simulink model "BESSV6_Switchmodel"  (R2020b)
settings: Solver=FixedStepDiscrete  StartTime=0.0  StopTime=10  FixedStep=Tplant  RelTol=1e-3
undefined symbols (not defined in the file): D1, DCL_LSC_LCL_Trafo_NoSwitching, Delta, DiscIntNeverNeededParam, dq_to_abc_single_dual, ess, Idq_Dec_Signs_Fdbk_Ref, pwrsysVICtrl, pwrsysVSrc, systemBase, Tplant
libraries: powerlib x54, pwrsysBasic x15, powerlib_meascontrol x14, pwrsysTransf x7, simulink x3
settings Model: Creator=lokaladm_josephkb  LastModifiedBy=josephkb
settings DataIOCC: ReturnWorkspaceOutputs=off
settings SFSimCC: CustomCodeUndefinedFunction=UseInterfaceOnly

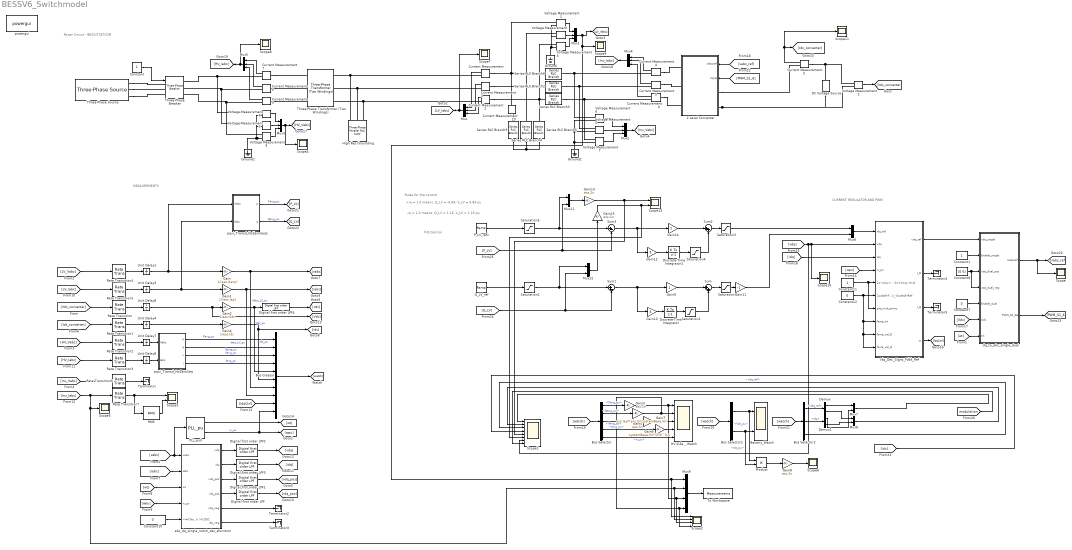
== system BESSV6_Switchmodel ==
  note: P-Q Control
  note: +iq = 1.0 means, Q_LV = -0.84, V_LV = 0.84 pu
  note: Rules for the control
  note: Power Circuit - BESS/STATCOM
  note: MEASUREMENTS
  note: CURRENT REGULATOR AND PWM
  note: -iq = 1.0 means, Q_LV = 1.16, V_LV = 1.16 pu
  2 Level Converter : Subsystem  AncestorBlock=pwrsysVSrc/DCL_LSC_LCL_Trafo_NoSwitching  mask(DCL + LSC + LCL + Trafo){Sn=ess.Sn, fn=systemBase.fn, Uhv_ab=systemBase.Vn, Uab=ess.Un, lf2=ess.LCL.l2, rf2=ess.LCL.r2, Lf1=ess.LCL.L1, Rf1=ess.LCL.R1, Cf=ess.LCL.Cf, Rc=ess.LCL.Rf, Cdc=ess.Cdc, Udc0=ess.Udc, Tsm=ess.Ts_control, Tstart=ess.DCVCont.Start}
      mask prompts: Sn "Rated apparent power [VA]"; fn "Rated frequency [Hz]"; Uhv_ab "Trafo HV rated line voltage [V]"; Uab "Trafo LV rated line voltage [V]"; lf2 "Trafo short-circuit inductance, lf2 [pu]"; rf2 "Trafo short-circuit resistance, rf2 [pu]"; Lf1 "Inverter side inductande, Lf1 [H]"; Rf1 "Inverter side parasitic resistance, Rf1 [Ohm]"; Cf "Shunt branch capacitance, Cf [F]"; Rc "Shunt branch damping resistance, Rc [Ohm]"; Cdc "DC-link shunt capacitance, Cdc [F]"; Udc0 "DC-link initial voltage [V]"; Tsm "Measurement sampling time [s]"; Tstart "Start time [s]"
      mask help:
      | DC Link + Line-side converter + LCL filter + Transformer
      |
      | DCL: current sources
      | 	Cdc: shunt capacitor of DC-link
      |
      | LSC: voltage source
      | 	fpwm: PWM frequency
      | LCL:
      | 	Lf1 + Rf1: inverter side reactor
      | 	Cf + Rc: shunt capacitor and damping resistor
      | 	Lf2 + Rf2: transformer short circuit inductance and resistance
      |
      | Transformer:	Y d1
      | 	HV: Y ungrounded
      | 	LV: delta
      |
      | High resistive grounding on LV side of tranformer (0.001W)
  Battery_Watch : Scope  NumInputPorts=2
  Bus Creator : BusCreator  Inputs=10
  Bus Selector : BusSelector  OutputSignals=Pavg_pu,Qavg_pu,Vavg_pu,Iavg_pu,w_pu
  Bus Selector1 : BusSelector  OutputSignals=Vdc_pu,Idc_pu
  Bus Selector2 : BusSelector  OutputSignals=IdqCtrl.Idq_ref,IdqCtrl.Idq,IdqCtrl.vdq_ref
  Constant : Constant
  Constant1 : Constant  SampleTime=ess.Ts_control
  Constant10 : Constant  Value=0  SampleTime=ess.Ts_control
  Constant11 : Constant  SampleTime=ess.Ts_control
  Constant12 : Constant  Value=0  SampleTime=ess.Ts_control
  Constant7 : Constant  Value=0  SampleTime=ess.Ts_control
  Constant9 : Constant  Value=[0 0]  SampleTime=ess.Ts_control
  Current Measurement{,1..10} (11 alike) : powerlib/Measurements/Current Measurement  PhasorSimulation=off  OutputType=Complex  PSBequivalent=0
  DC Voltage Source : powerlib/Electrical Sources/DC Voltage Source  Amplitude=ess.Udc  Measurements=None
  Demux : Demux  Outputs=2
  Demux1 : Demux  Outputs=2
  Digital first order LPF{,1..4} (5 alike) : pwrsysBasic/Digital first order LPF  Ts=ess.Ts_control  fcutout=ess.CurrCont.f_LPF_noise
      settings: SourceProductName=NTNU Power Systems
  Discrete-Time Integrator : DiscreteIntegrator  SampleTime=-1  ICPrevOutput=DiscIntNeverNeededParam  ICPrevScaledInput=DiscIntNeverNeededParam
  Discrete-Time Integrator1 : DiscreteIntegrator  SampleTime=-1  ICPrevOutput=DiscIntNeverNeededParam  ICPrevScaledInput=DiscIntNeverNeededParam
  Gain : Gain  Gain=1/(ess.Uanp)
  Gain1 : Gain  Gain=1/(ess.Iap)
  Gain10 : Gain  Gain=3
  Gain11 : Gain  Gain=-1
  Gain12 : Gain  Gain=3
  Gain{3,5,8,13,15} (5 alike) : Gain  Gain=ess.Sn
  Gain14 : Gain
  Gain2 : Gain  Gain=1/ess.Udc
  Gain4 : Gain  Gain=1/ess.Idc
  Gain6 : Gain  Gain=systemBase.Vn*(2/3)^0.5
  Gain7 : Gain  Gain=ess.Iap*(ess.Un/systemBase.Vn)
  Gain9 : Gain
  Ground : powerlib/Elements/Ground  LConnTagsString=a
  Ground1 : powerlib/Elements/Ground  LConnTagsString=a
  Ground2 : powerlib/Elements/Ground  LConnTagsString=a
  HV Side _ Watch : Scope  NumInputPorts=5
  High Res Grounding : powerlib/Elements/Three-Phase Parallel RLC Load  LConnTagsString=A|B|C  Configuration=Y (grounded)  NominalVoltage=ess.Un  Vabc=[1e3 1e3 1e3]  Vabcp=[1e3 1e3 1e3]  NominalFrequency=ess.Fn  UnbalancedPower=off  ActivePower=0.001  InductivePower=0  CapacitivePower=0  Pabc=[10e3 9e3 11e3]  QLabc=[100 90 110]  QCabc=[100 90 110]  Pabcp=[10e3 9e3 11e3]  QLabcp=[100 90 110]  QCabcp=[100 90 110]  Measurements=None  LoadType=constant Z
  Idq_Dec_Signs_Fdbk_Ref : Subsystem  AncestorBlock=pwrsysVICtrl/Idq_Dec_Signs_Fdbk_Ref  mask(Idq Controller - PI regulator with anti-windup){Ts=ess.Ts_control, fn=systemBase.fn, Kp=0.2, Ti=0.2/1, L=ess.CurrCont.x, PI_max=ess.CurrCont.PImax, PI_min=ess.CurrCont.PImin, TrafoPhaseComp=0}
      mask prompts: Ts "Sampling time [s]"; fn "Rated frequency: fn [Hz]"; Kp "Proportional gain: Kp [pu]"; Ti "Integral time: Ti [s]"; L "DQ decoupl. inductance: L [pu]"; PI_max "Maximum output [pu]"; PI_min "Minimum output [pu]"; TrafoPhaseComp "Transformer phase compensation [rad]"
      mask help:
      | Idq Controller
      | Discrete PI regulator with forward Euler approximation for the integrator.
      | Transfer function: 	Kp (1 + sTi) / (sTi)
      | The anti-windup freezes the integrator if the unlimited output of the PI goes beyond the limits.
      |
      | Phase compensation for transformer winding: PhaseTrafoComp
  Mux{,1..5} (6 alike) : Mux  Inputs=3
  Mux{6..8,11..12} (5 alike) : Mux  Inputs=2
  Mux9 : Mux
  PLL_pu3 : pwrsysBasic/PLL_pu  fn=systemBase.fn  Ts=ess.Ts_control  Kp_pll=90  Ki_pll=1200  Kd_pll=0  PLL_ini=60
      settings: SourceProductName=NTNU Power Systems
  P_LV_ref1 : simulink/Sources/Ramp  slope=0.5  start=2  InitialOutput=0
  Product : Product
  Q_LV_ref : simulink/Sources/Ramp  slope=0.2  start=15  InitialOutput=0
  RMS : powerlib_meascontrol/Measurements/RMS  TrueRMS=on  Freq=60  RMSInit=120  Ts=ess.Ts_control
  Rate Transition{,1..7} (8 alike) : RateTransition  OutPortSampleTime=ess.Ts_control
  Saturation{,1,3..4} (4 alike) : Saturate  UpperLimit=1  LowerLimit=-1
  Saturation2 : Saturate  UpperLimit=0.15  LowerLimit=-0.15
  Saturation5 : Saturate  LowerLimit=-0.4
  Scope{,4..11} (9 alike) : Scope
  Scope1 : Scope  NumInputPorts=8
  Scope13 : Scope  NumInputPorts=2
  Scope2 : Scope  NumInputPorts=4
  Scope3 : Scope  NumInputPorts=2
  Series RLC Branch2 : powerlib/Elements/Series RLC Branch  LConnTagsString=__new0  RConnTagsString=__new0  BranchType=RL  Resistance=ess.LCL.R1  Inductance=ess.LCL.L1  SetiL0=off  InitialCurrent=0  Capacitance=1e-6  Setx0=off  InitialVoltage=0  Measurements=None
  Series RLC Branch3 : powerlib/Elements/Series RLC Branch  LConnTagsString=__new0  RConnTagsString=__new0  BranchType=RL  Resistance=ess.LCL.R1  Inductance=ess.LCL.L1  SetiL0=off  InitialCurrent=0  Capacitance=1e-6  Setx0=off  InitialVoltage=0  Measurements=None
  Series RLC Branch4 : powerlib/Elements/Series RLC Branch  LConnTagsString=__new0  RConnTagsString=__new0  BranchType=RC  Resistance=ess.LCL.Rf  Inductance=1e-3  SetiL0=off  InitialCurrent=0  Capacitance=ess.LCL.Cf  Setx0=off  InitialVoltage=0  Measurements=None
  Series RLC Branch5 : powerlib/Elements/Series RLC Branch  LConnTagsString=__new0  RConnTagsString=__new0  BranchType=RC  Resistance=ess.LCL.Rf  Inductance=1e-3  SetiL0=off  InitialCurrent=0  Capacitance=ess.LCL.Cf  Setx0=off  InitialVoltage=0  Measurements=None
  Series RLC Branch6 : powerlib/Elements/Series RLC Branch  LConnTagsString=__new0  RConnTagsString=__new0  BranchType=RL  Resistance=ess.LCL.R1  Inductance=ess.LCL.L1  SetiL0=off  InitialCurrent=0  Capacitance=1e-6  Setx0=off  InitialVoltage=0  Measurements=None
  Series RLC Branch9 : powerlib/Elements/Series RLC Branch  LConnTagsString=__new0  RConnTagsString=__new0  BranchType=RC  Resistance=ess.LCL.Rf  Inductance=1e-3  SetiL0=off  InitialCurrent=0  Capacitance=ess.LCL.Cf  Setx0=off  InitialVoltage=0  Measurements=None
  Sum : Sum  Inputs=|++
  Sum1 : Sum  Inputs=|+-
  Sum2 : Sum  Inputs=|++
  Sum3 : Sum  Inputs=|+-
  Terminator{,2..5} (5 alike) : Terminator
  Three-Phase Transformer (Two Windings) : powerlib/Elements/Three-Phase Transformer (Two Windings)  Winding1Connection=Y  Winding2Connection=Delta (D1)  CoreType=Three single-phase transformers  SetSaturation=off  Hysteresis=off  DataFile='hysteresis'  SetInitialFlux=off  Measurements=None  UNITS=pu  NominalPower=[ess.Sn , ess.Fn]  Winding1=[systemBase.Vn ess.LCL.r2 ess.LCL.l2]  Winding2=[ess.Un ess.LCL.r2 ess.LCL.l2]  Rm=500.01  Lm=416.67  L0=0.5  Saturation=[0 0;0.0024 1;0.99999 1.2667]  InitialFluxes=[0.80002 -0.80002 0.7]  BreakLoop=off  DiscreteSolver=Trapezoidal iterative  DataType=off  TransfoNumber=1
  Three-Phase Breaker : powerlib/Elements/Three-Phase Breaker  InitialState=open  SwitchA=on  SwitchB=on  SwitchC=on  SwitchTimes="[1/60  5/60]"  External=on  BreakerResistance=0.01  SnubberResistance=1e6  SnubberCapacitance=1e9  Measurements=None
  Three-Phase Source : powerlib/Electrical Sources/Three-Phase Source  InternalConnection=Yg  VoltagePhases=off  Voltage=systemBase.Vn  PhaseAngle=0  Voltage_phases=[25e3 25e3 25e3]/sqrt(3)  PhaseAngles_phases=[0 -120 +120]  Frequency=systemBase.fn  NonIdealSource=on  SpecifyImpedance=off  Resistance=5e-3  Inductance=0.2e-6  ShortCircuitLevel=SCMVA  BaseVoltage=systemBase.Vn  XRratio=X_R  BusType=swing  Pref=10e3  Qref=0  Prefabc=[10e3, 10e3, 10e3]  Qrefabc=[0, 0, 0]  Qmin=-inf  Qmax=inf
  To Workspace : ToWorkspace  VariableName=Measurements  SaveFormat=Structure With Time  SampleTime=ess.Ts_control
  Unit Delay{1,3,7..8} (4 alike) : UnitDelay  InitialCondition=[0 0 0]  SampleTime=ess.Ts_control  HasFrameUpgradeWarning=on
  Unit Delay4 : UnitDelay  SampleTime=ess.Ts_control  HasFrameUpgradeWarning=on
  Unit Delay6 : UnitDelay  InitialCondition=1  SampleTime=ess.Ts_control  HasFrameUpgradeWarning=on
  Voltage Measurement{,1..9} (10 alike) : powerlib/Measurements/Voltage Measurement  PhasorSimulation=off  OutputType=Complex  PSBequivalent=0
  abc_dq_single_notch_dsc_sfunction : Subsystem  AncestorBlock=pwrsysTransf/abc_dq_single_notch_dsc_sfunction  mask(abc->dq with Matlab){Ts=ess.Ts_control, fn=2*systemBase.fn, zeta=ess.CurrCont.zeta}
      mask prompts: Ts "Sampling time [s]"; fn "Notch frequency [Hz]"; zeta "Zeta for notch filters"
      mask help:
      | To be done
      |
      | Max buffer size for DSC 500 samples
  dq_to_abc_single_dual : Subsystem  AncestorBlock=pwrsysVICtrl/dq_to_abc_single_dual  mask(Scaling of vdq ref and PWM gate generation){Ts=ess.Ts_control, Uabp=ess.Uabp}
      mask prompts: Ts "Sampling time [s]"; Uabp "Rated peak line voltage [V]"
      mask help:
      | Scales vdq_ref by: U_line_peak / Udc
      |
      | Add third harmonic to uabc_ref for overmodulation
  powergui : powerlib/powergui  Priority=1  SimulationMode=Discrete  SampleTime=Tplant  frequency=60  Iterations=50  frequencyindice=0  Pbase=100e6  ErrMax=1e-4  UnitsV=kV  UnitsW=MW  buscounter=0  FunctionMessages=off  echomessages=off  EnableUseOfTLC=off  CurrentSourceSwitches=off  DisableSnubberDevices=off  DisableRonSwitches=off  DisableVfSwitches=off  DisplayEquations=off  AutomaticDiscreteSolvers=off  SolverType=Tustin/Backward Euler (TBE)  Interpol=off  ExternalGateDelay=off  methode=off  Ts=100  x0status=blocks  SPID=on  SwTol=0  HookPort=off  NonlinearTolerance=0  nMaxIteration=15  ContinueOnMaxIteration=off  RestoreLinks=warning  ResistiveCurrentMeasurement=off  Frange=[0:2:500]  Ylog=off  Xlog=on  ShowGrid=off  save=off  variable=ZData  structure=0  ZoomFFT=off  StartTime=0.0  cycles=1  DisplayStyle=1  fundamental=60  FreqAxis=off  MaxFrequency=1000  frequencyindicesteady=1  RmsSteady=1  display=off
  pqui_Transd_NoZeroSeq : Subsystem  AncestorBlock=pwrsysBasic/pqui_Transd_NoZeroSeq  mask(u i p q transducer - No zero sequence){Sn=ess.Sn, Uanp=systemBase.Vn*(2/3)^0.5, Iap=ess.Iap*(ess.Un/systemBase.Vn)}
      mask prompts: Sn "Rated three-phase apparent power [VA]"; Uanp "Rated peak phase-to-groud voltage [V]"; Iap "Rated peak line current [A]"
      mask help:
      | Loosely based on Akagi 1984, but with Clarke Transformation for both the current and voltage
      | 	v  = (valpha^2 + vbeta^2)^0.5 / V_phase_peak
      | 	i   = (ialpha^2 + ibeta^2)^0.5 / I_line_peak
      | 	p  = 3/2 * (valpha ialpha +vbeta ibeta) / Sn
      | 	q  = 3/2 * (-valpha ibeta +vbeta ialpha) / Sn
  pqui_Transd_NoZeroSeq1 : Subsystem  AncestorBlock=pwrsysBasic/pqui_Transd_NoZeroSeq  mask(u i p q transducer - No zero sequence){Sn=ess.Sn, Uanp=systemBase.Vn*(2/3)^0.5, Iap=ess.Iap*(ess.Un/systemBase.Vn)}
      mask prompts: Sn "Rated three-phase apparent power [VA]"; Uanp "Rated peak phase-to-groud voltage [V]"; Iap "Rated peak line current [A]"
      mask help:
      | Loosely based on Akagi 1984, but with Clarke Transformation for both the current and voltage
      | 	v  = (valpha^2 + vbeta^2)^0.5 / V_phase_peak
      | 	i   = (ialpha^2 + ibeta^2)^0.5 / I_line_peak
      | 	p  = 3/2 * (valpha ialpha +vbeta ibeta) / Sn
      | 	q  = 3/2 * (-valpha ibeta +vbeta ialpha) / Sn
  wires:
  Voltage Measurement2/1 -> [Vdc_converter]
  Mux/1 -> Scope7/1, [LV_Iabc]
  Voltage Measurement/1 -> Mux1/2
  Voltage Measurement1/1 -> Mux1/1
  Voltage Measurement4/1 -> Mux1/3
  Mux1/1 -> Scope2/1, Mux9/1, Scope9/1, [LV_Vabc]
  Mux2/1 -> [Inv_Vabc]
  Voltage Measurement6/1 -> Mux2/1
  Voltage Measurement7/1 -> Mux2/3
  Voltage Measurement5/1 -> Mux2/2
  Current Measurement/1 -> Mux/1
  Current Measurement1/1 -> Mux/2
  Current Measurement2/1 -> Mux/3
  [iabc] -> abc_dq_single_notch_dsc_sfunction/2(iabc)
  pqui_Transd_NoZeroSeq/4(i) -> Bus Creator/4  "Iavg_pu"
  Digital first order LPF3/1 -> [idq]
  Digital first order LPF/1 -> [idq_pos]
  abc_dq_single_notch_dsc_sfunction/4(idq_pos) -> Digital first order LPF/1
  Digital first order LPF2/1 -> [vdq]
  Bus Creator/1 -> [watch]
  Unit Delay3/1 -> pqui_Transd_NoZeroSeq1/2(Iabc), Gain1/1
  abc_dq_single_notch_dsc_sfunction/1(vdq) -> Digital first order LPF2/1
  Digital first order LPF4/1 -> [vdc]
  abc_dq_single_notch_dsc_sfunction/2(idq) -> Digital first order LPF3/1
  [vabc] -> abc_dq_single_notch_dsc_sfunction/1(vabc), PLL_pu3/1
  Unit Delay8/1 -> pqui_Transd_NoZeroSeq/2(Iabc)
  abc_dq_single_notch_dsc_sfunction/3(vdq_pos) -> Digital first order LPF1/1
  Gain1/1 -> [iabc], Bus Creator/8  "Iabc_LV_pu"
  [wt] -> abc_dq_single_notch_dsc_sfunction/3(wt)
  [wpu] -> abc_dq_single_notch_dsc_sfunction/4(w_pu)
  Unit Delay6/1 -> [Vdc], Gain2/1
  Unit Delay7/1 -> pqui_Transd_NoZeroSeq/1(Vabc)
  abc_dq_single_notch_dsc_sfunction/6(idq_neg) -> Terminator3/1
  Gain2/1 -> Digital first order LPF4/1, Bus Creator/5  "Vdc_pu"
  Unit Delay1/1 -> pqui_Transd_NoZeroSeq1/1(Vabc), Gain/1
  PLL_pu3/1 -> [wt]
  abc_dq_single_notch_dsc_sfunction/5(vdq_neg) -> Terminator2/1
  Unit Delay4/1 -> Gain4/1
  Rate Transition2/1 -> Unit Delay7/1
  Rate Transition/1 -> Unit Delay6/1
  pqui_Transd_NoZeroSeq/1(p) -> Bus Creator/1  "Pavg_pu"
  PLL_pu3/2 -> Bus Creator/10, [wpu]  "w_pu"
  Rate Transition1/1 -> Unit Delay4/1
  [IdqCtrl] -> Bus Creator/9
  Digital first order LPF1/1 -> [vdq_pos]
  pqui_Transd_NoZeroSeq/3(v) -> Bus Creator/3  "Vavg_pu"
  Gain/1 -> [vabc], Bus Creator/7  "Vabc_LV_pu"
  Rate Transition3/1 -> Unit Delay8/1
  Gain4/1 -> [idc], Bus Creator/6  "Idc_pu"
  Constant10/1 -> abc_dq_single_notch_dsc_sfunction/5(<=0:Notch,>0:DSC)
  Rate Transition5/1 -> Unit Delay3/1
  Rate Transition4/1 -> Unit Delay1/1
  pqui_Transd_NoZeroSeq/2(q) -> Bus Creator/2  "Qavg_pu"
  Current Measurement3/1 -> Scope11/1, [Idc_converter]
  Voltage Measurement9/1 -> Mux3/3
  Voltage Measurement3/1 -> Mux3/2
  Voltage Measurement8/1 -> Mux3/1
  Constant/1 -> Three-Phase Breaker/1
  Current Measurement7/1 -> Mux5/1
  Current Measurement8/1 -> Mux5/2
  Mux5/1 -> Scope8/1, [HV_Iabc]
  Current Measurement9/1 -> Mux5/3
  Mux4/1 -> [Inv_Iabc]
  Current Measurement4/1 -> Mux4/1
  Current Measurement5/1 -> Mux4/2
  Current Measurement6/1 -> Mux4/3
  [Vdc_converter] -> Rate Transition/1
  [Idc_converter] -> Rate Transition1/1
  [HV_Vabc] -> Rate Transition2/1
  [HV_Iabc] -> Rate Transition3/1
  [LV_Vabc] -> Rate Transition4/1
  [LV_Iabc] -> Rate Transition5/1
  [Inv_Vabc] -> Rate Transition6/1
  [Inv_Iabc] -> Scope2/2, Mux9/2, Scope5/1, Rate Transition7/1
  Rate Transition6/1 -> Terminator/1
  Rate Transition7/1 -> RMS/1, Scope3/1
  [wpu] -> Idq_Dec_Signs_Fdbk_Ref/4(w_pu)
  Constant12/1 -> Idq_Dec_Signs_Fdbk_Ref/8(force_int), Idq_Dec_Signs_Fdbk_Ref/9(force_val_D), Idq_Dec_Signs_Fdbk_Ref/10(force_val_Q), Idq_Dec_Signs_Fdbk_Ref/6(1=decFrFbk_-0=decFrRef)
  Idq_Dec_Signs_Fdbk_Ref/3(I_Q) -> Terminator5/1
  Idq_Dec_Signs_Fdbk_Ref/4(m) -> [IdqCtrl]
  Constant11/1 -> Idq_Dec_Signs_Fdbk_Ref/7(pre_mult_errors), Idq_Dec_Signs_Fdbk_Ref/5(1=-wLiq,+wLid_-1=+wLiq,-wLid)
  [vdq] -> Scope1/7, Scope10/1, Idq_Dec_Signs_Fdbk_Ref/2(vdq)
  Constant9/1 -> dq_to_abc_single_dual/4(vdq_dual_neg), dq_to_abc_single_dual/3(vdq_dual_pos)
  Constant1/1 -> dq_to_abc_single_dual/2(Enable_single)
  Constant7/1 -> dq_to_abc_single_dual/5(Enable_dual)
  [wt] -> dq_to_abc_single_dual/7(wt)
  Idq_Dec_Signs_Fdbk_Ref/2(I_D) -> Terminator4/1
  [Vdc] -> dq_to_abc_single_dual/6(Udc)
  dq_to_abc_single_dual/1(Uabcref) -> Scope/1, [vabc_ref]
  [idq] -> Idq_Dec_Signs_Fdbk_Ref/3(idq)
  Idq_Dec_Signs_Fdbk_Ref/1(vdq_ref) -> dq_to_abc_single_dual/1(vdq_single)
  Mux6/1 -> Idq_Dec_Signs_Fdbk_Ref/1(idq_ref)
  [vabc_ref] -> 2 Level Converter/1(Vabcref)
  [watch] -> Bus Selector/1
  Bus Selector/1 -> Gain3/1  "<Pavg_pu>"
  Bus Selector/2 -> Gain5/1  "<Qavg_pu>"
  Bus Selector/3 -> Gain6/1  "<Vavg_pu>"
  Bus Selector/4 -> Gain7/1  "<Iavg_pu>"
  Bus Selector/5 -> HV Side _ Watch/5  "<w_pu>"
  Bus Selector1/1 -> Product/1, Battery_Watch/1  "<Vdc_pu>"
  Bus Selector1/2 -> Product/2, Battery_Watch/2  "<Idc_pu>"
  [watch] -> Bus Selector1/1
  [watch] -> Bus Selector2/1
  Bus Selector2/1 -> Demux/1  "<Idq_ref>"
  Bus Selector2/2 -> Demux1/1  "<Idq>"
  Bus Selector2/3 -> Scope1/3  "<vdq_ref>"
  Mux7/1 -> Scope1/1
  Mux8/1 -> Scope1/2
  Demux/1 -> Mux7/1
  Demux1/1 -> Mux7/2
  Demux/2 -> Mux8/1
  Demux1/2 -> Mux8/2
  [idc] -> Scope1/4
  RMS/1 -> Scope3/2
  Gain3/1 -> Scope2/3, Mux9/3, HV Side _ Watch/1
  Gain5/1 -> Scope2/4, Mux9/4, HV Side _ Watch/2
  Gain6/1 -> HV Side _ Watch/3
  Gain7/1 -> HV Side _ Watch/4
  Product/1 -> Gain8/1
  Gain8/1 -> Scope6/1
  Mux3/1 -> Scope4/1, [HV_Vabc]
  pqui_Transd_NoZeroSeq1/1(p) -> [P_LV]  "Pavg_pu"
  Gain10/1 -> Discrete-Time Integrator/1
  Discrete-Time Integrator/1 -> Saturation1/1
  Sum/1 -> Saturation/1
  Gain9/1 -> Sum/1
  Saturation1/1 -> Sum/2
  Sum1/1 -> Gain10/1, Gain9/1
  Q_LV_ref/1 -> Saturation2/1
  Mux12/1 -> Gain15/1
  Saturation/1 -> Gain11/1
  Gain11/1 -> Mux6/2
  Saturation2/1 -> Mux12/1, Sum1/1
  pqui_Transd_NoZeroSeq1/2(q) -> [Q_LV]  "Qavg_pu"
  [Q_LV] -> Mux12/2, Sum1/2
  Sum2/1 -> Saturation3/1
  Sum3/1 -> Gain12/1, Gain14/1
  Gain14/1 -> Sum2/1
  Mux11/1 -> Gain13/1
  Gain12/1 -> Discrete-Time Integrator1/1
  Discrete-Time Integrator1/1 -> Saturation4/1
  [P_LV] -> Sum3/2, Mux11/2
  P_LV_ref1/1 -> Saturation5/1
  Saturation5/1 -> Mux11/1, Sum3/1
  Saturation4/1 -> Sum2/2
  Saturation3/1 -> Mux6/1
  Gain13/1 -> Scope1/5, Scope13/1
  Gain15/1 -> Scope1/6, Scope13/2
  [modulation] -> Scope1/8
  dq_to_abc_single_dual/2(PWM_S1_S6) -> [PWM_S1_6]
  [PWM_S1_6] -> 2 Level Converter/2(PWM)
  Mux9/1 -> To Workspace/1
  connections:
  Voltage Measurement3/LConn1 -- Current Measurement8/RConn1 -- Three-Phase Breaker/RConn2
  Three-Phase Breaker/RConn1 -- Current Measurement7/RConn1 -- Voltage Measurement8/LConn1
  Voltage Measurement9/LConn1 -- Current Measurement9/RConn1 -- Three-Phase Breaker/RConn3
  Current Measurement/RConn1 -- Three-Phase Transformer (Two Windings)/RConn1 -- High Res Grounding/LConn1
  Series RLC Branch6/LConn1 -- Voltage Measurement1/LConn1 -- Current Measurement/LConn1 -- Current Measurement10/LConn1
  Series RLC Branch4/LConn1 -- Series RLC Branch2/LConn1 -- Current Measurement1/LConn1 -- Voltage Measurement/LConn1
  Series RLC Branch5/LConn1 -- Series RLC Branch3/LConn1 -- Current Measurement2/LConn1 -- Voltage Measurement4/LConn1
  Current Measurement1/RConn1 -- Three-Phase Transformer (Two Windings)/RConn2 -- High Res Grounding/LConn2
  Current Measurement2/RConn1 -- Three-Phase Transformer (Two Windings)/RConn3 -- High Res Grounding/LConn3
  Voltage Measurement2/LConn1 -- Current Measurement3/LConn1 -- DC Voltage Source/RConn1
  2 Level Converter/LConn2 -- DC Voltage Source/LConn1 -- Voltage Measurement2/LConn2
  Ground/LConn1 -- Voltage Measurement4/LConn2 -- Voltage Measurement/LConn2 -- Voltage Measurement1/LConn2
  Series RLC Branch6/RConn1 -- Current Measurement4/RConn1 -- Voltage Measurement6/LConn1
  Series RLC Branch2/RConn1 -- Current Measurement5/RConn1 -- Voltage Measurement5/LConn1
  Series RLC Branch3/RConn1 -- Current Measurement6/RConn1 -- Voltage Measurement7/LConn1
  2 Level Converter/LConn1 -- Current Measurement3/RConn1
  Voltage Measurement9/LConn2 -- Ground1/LConn1 -- Voltage Measurement3/LConn2 -- Voltage Measurement8/LConn2
  Three-Phase Source/RConn1 -- Three-Phase Breaker/LConn1
  Three-Phase Source/RConn2 -- Three-Phase Breaker/LConn2
  Three-Phase Source/RConn3 -- Three-Phase Breaker/LConn3
  Current Measurement7/LConn1 -- Three-Phase Transformer (Two Windings)/LConn1
  Current Measurement8/LConn1 -- Three-Phase Transformer (Two Windings)/LConn2
  Current Measurement9/LConn1 -- Three-Phase Transformer (Two Windings)/LConn3
  Series RLC Branch5/RConn1 -- Series RLC Branch9/RConn1 -- Series RLC Branch4/RConn1
  Voltage Measurement6/LConn2 -- Voltage Measurement5/LConn2 -- Voltage Measurement7/LConn2 -- Ground2/LConn1
  Current Measurement4/LConn1 -- 2 Level Converter/RConn1
  Current Measurement5/LConn1 -- 2 Level Converter/RConn2
  Current Measurement6/LConn1 -- 2 Level Converter/RConn3
  Current Measurement10/RConn1 -- Series RLC Branch9/LConn1

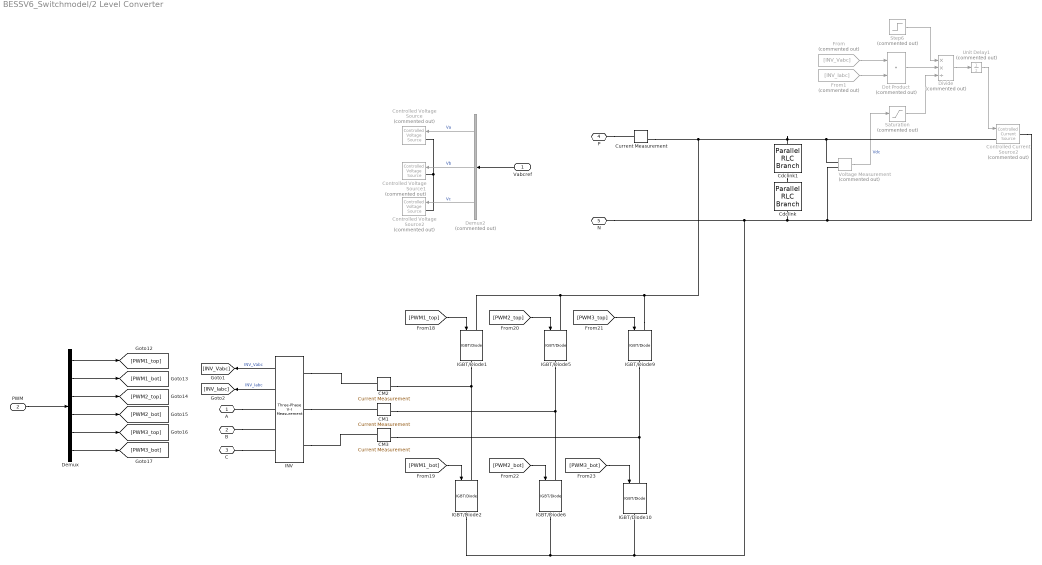
== system BESSV6_Switchmodel/2 Level Converter ==
  Vabcref : Inport
  PWM : Inport  Port=2
  CM1 : powerlib/Measurements/Current Measurement  PhasorSimulation=off  OutputType=Complex  PSBequivalent=0
  CM2 : powerlib/Measurements/Current Measurement  PhasorSimulation=off  OutputType=Complex  PSBequivalent=0
  CM3 : powerlib/Measurements/Current Measurement  PhasorSimulation=off  OutputType=Complex  PSBequivalent=0
  Cdclink : powerlib/Elements/Parallel RLC Branch  LConnTagsString=a  RConnTagsString=__new0  BranchType=RC  Resistance=1e6  Inductance=0  SetiL0=off  InitialCurrent=0  Capacitance=Cdc  Setx0=on  InitialVoltage=Udc0  Measurements=None
  Cdclink1 : powerlib/Elements/Parallel RLC Branch  LConnTagsString=a  RConnTagsString=__new0  BranchType=R  Resistance=1e-3  Inductance=0  SetiL0=off  InitialCurrent=0  Capacitance=Cdc  Setx0=on  InitialVoltage=Udc0  Measurements=None
  Controlled Current Source2 : powerlib/Electrical Sources/Controlled Current Source  Commented=on  Initialize=on  Source_Type=DC  Amplitude=0  Phase=0  Frequency=50  Measurements=None
  Controlled Voltage Source : powerlib/Electrical Sources/Controlled Voltage Source  Commented=on  Initialize=on  Source_Type=AC  Amplitude=Uab*(2/3)^0.5  Phase=30  Frequency=fn  Measurements=None
  Controlled Voltage Source1 : powerlib/Electrical Sources/Controlled Voltage Source  Commented=on  Initialize=on  Source_Type=AC  Amplitude=Uab*(2/3)^0.5  Phase=30-120  Frequency=fn  Measurements=None
  Controlled Voltage Source2 : powerlib/Electrical Sources/Controlled Voltage Source  Commented=on  Initialize=on  Source_Type=AC  Amplitude=Uab*(2/3)^0.5  Phase=30+120  Frequency=fn  Measurements=None
  Current Measurement : powerlib/Measurements/Current Measurement  PhasorSimulation=off  OutputType=Complex  PSBequivalent=0
  Demux : Demux  Outputs=6
  Demux2 : Demux  Commented=on  Outputs=3
  Divide : Product  Commented=on  Inputs=**/
  Dot Product : DotProduct  Commented=on  InputSameDT=on  OutDataTypeStr=Inherit: Inherit via internal rule
  From : From  Commented=on  GotoTag=INV_Vabc
  From1 : From  Commented=on  GotoTag=INV_Iabc
  IGBT/Diode{1..2,5..6,9..10} (6 alike) : powerlib/Power Electronics/IGBT//Diode  Ron=1e-3  Rs=1e5  Cs=inf  Measurements=off
  INV : powerlib/Measurements/Three-Phase V-I Measurement  VoltageMeasurement=phase-to-ground  SetLabelV=off  LabelV=vconv  Vpu=off  VpuLL=off  CurrentMeasurement=yes  SetLabelI=off  LabelI=iconv  Ipu=off  Pbase=sn  Vbase=uab  OutputType=Complex  PhasorSimulation=off  PSBequivalent=0
  Saturation : Saturate  Commented=on  UpperLimit=10*Uab*sqrt(2/3)  LowerLimit=0.01*Uab*sqrt(2/3)
  Step6 : Step  Commented=on  Time=Tstart  SampleTime=Tsm
  Unit Delay1 : UnitDelay  Commented=on  SampleTime=Tsm  HasFrameUpgradeWarning=on
  Voltage Measurement : powerlib/Measurements/Voltage Measurement  Commented=on  PhasorSimulation=off  OutputType=Magnitude  PSBequivalent=0
  A : PMIOPort  Side=Right
  B : PMIOPort  Port=2  Side=Right
  C : PMIOPort  Port=3  Side=Right
  P : PMIOPort  Port=4  Side=Left
  N : PMIOPort  Port=5  Side=Left
  wires:
  Step6/1 -> Divide/1
  Unit Delay1/1 -> Controlled Current Source2/1
  From1/1 -> Dot Product/2
  From/1 -> Dot Product/1
  Divide/1 -> Unit Delay1/1
  Dot Product/1 -> Divide/2
  Saturation/1 -> Divide/3
  Voltage Measurement/1 -> Saturation/1  "Vdc"
  Demux2/3 -> Controlled Voltage Source2/1  "Vc"
  Demux2/2 -> Controlled Voltage Source1/1  "Vb"
  Demux2/1 -> Controlled Voltage Source/1  "Va"
  Vabcref/1 -> Demux2/1
  INV/2 -> [INV_Iabc]  "INV_Iabc"
  INV/1 -> [INV_Vabc]  "INV_Vabc"
  Demux/6 -> [PWM3_bot]
  Demux/1 -> [PWM1_top]
  Demux/2 -> [PWM1_bot]
  Demux/3 -> [PWM2_top]
  Demux/4 -> [PWM2_bot]
  Demux/5 -> [PWM3_top]
  PWM/1 -> Demux/1
  [PWM2_top] -> IGBT/Diode5/1
  [PWM3_bot] -> IGBT/Diode10/1
  [PWM3_top] -> IGBT/Diode9/1
  [PWM2_bot] -> IGBT/Diode6/1
  [PWM1_bot] -> IGBT/Diode2/1
  [PWM1_top] -> IGBT/Diode1/1
  connections:
  P/RConn1 -- Current Measurement/LConn1
  IGBT/Diode9/LConn1 -- Current Measurement/RConn1 -- Cdclink1/LConn1 -- Voltage Measurement/LConn1 -- Controlled Current Source2/LConn1 -- IGBT/Diode5/LConn1 -- IGBT/Diode1/LConn1
  IGBT/Diode10/RConn1 -- N/RConn1 -- Cdclink/RConn1 -- Controlled Current Source2/RConn1 -- Voltage Measurement/LConn2 -- IGBT/Diode6/RConn1 -- IGBT/Diode2/RConn1
  Controlled Voltage Source1/LConn1 -- Controlled Voltage Source/LConn1 -- Controlled Voltage Source2/LConn1
  C/RConn1 -- INV/RConn3
  B/RConn1 -- INV/RConn2
  A/RConn1 -- INV/RConn1
  Cdclink1/RConn1 -- Cdclink/LConn1
  CM1/RConn1 -- IGBT/Diode6/LConn1 -- IGBT/Diode5/RConn1
  CM3/RConn1 -- IGBT/Diode10/LConn1 -- IGBT/Diode9/RConn1
  CM2/RConn1 -- IGBT/Diode2/LConn1 -- IGBT/Diode1/RConn1
  INV/LConn1 -- CM2/LConn1
  INV/LConn2 -- CM1/LConn1
  INV/LConn3 -- CM3/LConn1

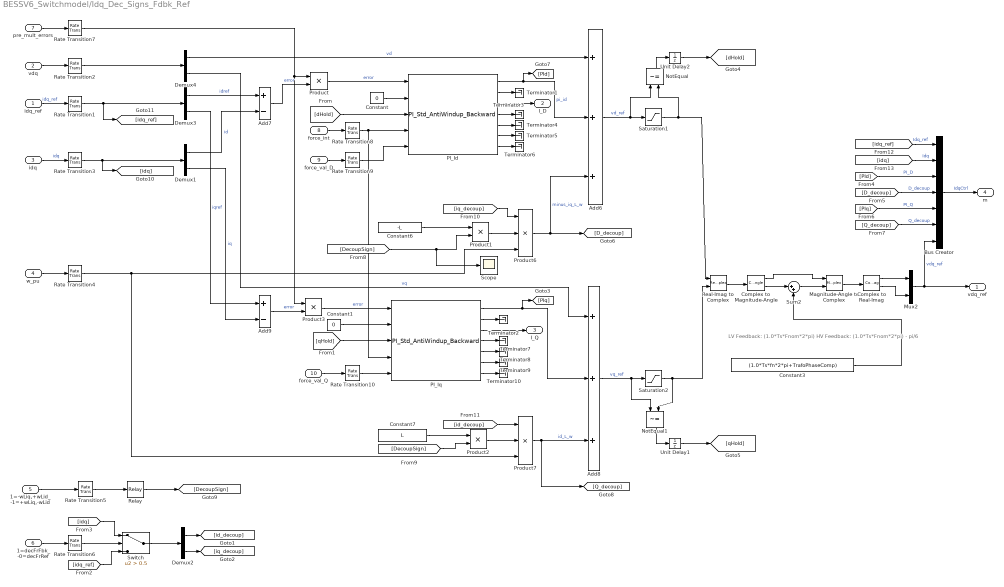
== system BESSV6_Switchmodel/Idq_Dec_Signs_Fdbk_Ref ==
  note: LV Feedback: (1.0*Ts*Fnom*2*pi)
      | HV Feedback: (1.0*Ts*Fnom*2*pi) - pi/6
  idq_ref : Inport
  vdq : Inport  Port=2
  idq : Inport  Port=3
  w_pu : Inport  Port=4
  1=-wLiq,+wLid_-1=+wLiq,-wLid : Inport  Port=5
  1=decFrFbk_-0=decFrRef : Inport  Port=6
  pre_mult_errors : Inport  Port=7
  force_int : Inport  Port=8
  force_val_D : Inport  Port=9
  force_val_Q : Inport  Port=10
  Add6 : Sum  Inputs=+++
  Add7 : Sum  Inputs=+-
  Add8 : Sum  Inputs=+++
  Add9 : Sum  Inputs=+-
  Bus Creator : BusCreator  Inputs=7
  Complex to Magnitude-Angle : ComplexToMagnitudeAngle
  Complex to Real-Imag : ComplexToRealImag
  Constant : Constant  Value=0  SampleTime=Ts
  Constant1 : Constant  Value=0  SampleTime=Ts
  Constant3 : Constant  Value=(1.0*Ts*fn*2*pi+TrafoPhaseComp)  SampleTime=Ts
  Constant6 : Constant  Value=-L  SampleTime=Ts
  Constant7 : Constant  Value=L  SampleTime=Ts
  Demux{1..4} (4 alike) : Demux  Outputs=2
  Magnitude-Angle to Complex : MagnitudeAngleToComplex
  Mux2 : Mux  Inputs=2
  NotEqual : RelationalOperator  Operator=~=  OutDataTypeStr=boolean  RndMeth=Nearest
  NotEqual1 : RelationalOperator  Operator=~=  OutDataTypeStr=boolean  RndMeth=Nearest
  PI_Id : pwrsysBasic/PI_Std_AntiWindup_Backward  Ts=Ts  Kg=Kp  Kp=1  Ti=Ti  outMax=PI_max  outMin=PI_min
      link override S-Function Builder: Parameters=Ts,Kg,Kp,Ti,outMax,outMin  FunctionName=pi_std_antiwindup
      settings: SourceProductName=NTNU Power Systems
  PI_Iq : pwrsysBasic/PI_Std_AntiWindup_Backward  Ts=Ts  Kg=Kp  Kp=1  Ti=Ti  outMax=PI_max  outMin=PI_min
      settings: SourceProductName=NTNU Power Systems
  Product : Product
  Product1 : Product  RndMeth=Zero
  Product2 : Product  RndMeth=Zero
  Product3 : Product
  Product6 : Product  Inputs=3  RndMeth=Zero
  Product7 : Product  Inputs=3  RndMeth=Zero
  Rate Transition1 : RateTransition  InitialCondition=[0 0]  OutPortSampleTime=Ts
  Rate Transition{6..10} (5 alike) : RateTransition  OutPortSampleTime=Ts
  Rate Transition2 : RateTransition  InitialCondition=[0 0]  OutPortSampleTime=Ts
  Rate Transition3 : RateTransition  InitialCondition=[0 0]  OutPortSampleTime=Ts
  Rate Transition4 : RateTransition  InitialCondition=1  OutPortSampleTime=Ts
  Rate Transition5 : RateTransition  InitialCondition=1  OutPortSampleTime=Ts
  Real-Imag to Complex : RealImagToComplex
  Relay : Relay  OnSwitchValue=0  OffSwitchValue=-0.1  OffOutputValue=-1
  Saturation1 : Saturate  UpperLimit=PI_max  LowerLimit=PI_min
  Saturation2 : Saturate  UpperLimit=PI_max  LowerLimit=PI_min
  Scope : Scope
  Sum2 : Sum  Inputs=|++
  Switch : Switch  Criteria=u2 > Threshold  Threshold=0.5
  Terminator{1..10} (10 alike) : Terminator
  Unit Delay1 : UnitDelay  SampleTime=Ts  HasFrameUpgradeWarning=on
  Unit Delay2 : UnitDelay  SampleTime=Ts  HasFrameUpgradeWarning=on
  vdq_ref : Outport
  I_D : Outport  Port=2
  I_Q : Outport  Port=3
  m : Outport  Port=4
  wires:
  Rate Transition10/1 -> PI_Iq/5
  Rate Transition9/1 -> PI_Id/5
  Rate Transition8/1 -> PI_Id/4, PI_Iq/4
  Rate Transition7/1 -> Product/1, Product3/1
  Rate Transition6/1 -> Switch/2
  Rate Transition5/1 -> Relay/1
  Rate Transition4/1 -> Product6/3, Product7/3
  Rate Transition3/1 -> [idq], Demux1/1
  Rate Transition1/1 -> Demux3/1, [idq_ref]
  Rate Transition2/1 -> Demux4/1
  Constant1/1 -> PI_Iq/2
  PI_Iq/1 -> [PIq], Add8/2
  PI_Iq/3 -> I_Q/1
  PI_Iq/7 -> Terminator10/1
  PI_Iq/6 -> Terminator9/1
  PI_Iq/5 -> Terminator8/1
  PI_Iq/4 -> Terminator7/1
  PI_Iq/2 -> Terminator2/1
  PI_Id/7 -> Terminator6/1
  PI_Id/6 -> Terminator5/1
  PI_Id/5 -> Terminator4/1
  PI_Id/4 -> Terminator3/1
  PI_Id/2 -> Terminator1/1
  Constant/1 -> PI_Id/2
  PI_Id/3 -> I_D/1
  pre_mult_errors/1 -> Rate Transition7/1
  Add7/1 -> Product/2  "error"
  Add9/1 -> Product3/2  "error"
  force_val_Q/1 -> Rate Transition10/1
  force_val_D/1 -> Rate Transition9/1
  force_int/1 -> Rate Transition8/1
  [idq] -> Bus Creator/2  "Idq"
  [idq_ref] -> Bus Creator/1  "Idq_ref"
  [id_decoup] -> Product7/1
  [iq_decoup] -> Product6/1
  [idq] -> Switch/1
  Switch/1 -> Demux2/1
  Demux2/1 -> [id_decoup]
  1=decFrFbk_-0=decFrRef/1 -> Rate Transition6/1
  Demux2/2 -> [iq_decoup]
  [idq_ref] -> Switch/3
  [DecoupSign] -> Product2/2
  Product2/1 -> Product7/2
  Product1/1 -> Product6/2
  [DecoupSign] -> Scope/1, Product1/2
  1=-wLiq,+wLid_-1=+wLiq,-wLid/1 -> Rate Transition5/1
  Relay/1 -> [DecoupSign]
  [qHold] -> PI_Iq/3
  [dHold] -> PI_Id/3
  Unit Delay1/1 -> [qHold]
  Unit Delay2/1 -> [dHold]
  NotEqual1/1 -> Unit Delay1/1
  Saturation2/1 -> Real-Imag to Complex/2, NotEqual1/2
  NotEqual/1 -> Unit Delay2/1
  Saturation1/1 -> Real-Imag to Complex/1, NotEqual/2
  [Q_decoup] -> Bus Creator/6  "Q_decoup"
  Bus Creator/1 -> m/1  "IdqCtrl"
  [PIq] -> Bus Creator/5  "PI_Q"
  [D_decoup] -> Bus Creator/4  "D_decoup"
  [PId] -> Bus Creator/3  "PI_D"
  Complex to Real-Imag/2 -> Mux2/2
  Complex to Real-Imag/1 -> Mux2/1
  Constant3/1 -> Sum2/2
  Sum2/1 -> Magnitude-Angle to Complex/2
  Complex to Magnitude-Angle/2 -> Sum2/1
  Complex to Magnitude-Angle/1 -> Magnitude-Angle to Complex/1
  Real-Imag to Complex/1 -> Complex to Magnitude-Angle/1
  Magnitude-Angle to Complex/1 -> Complex to Real-Imag/1
  Demux3/2 -> Add9/1  "iqref"
  Demux3/1 -> Add7/1  "idref"
  idq_ref/1 -> Rate Transition1/1  "idq_ref"
  Add6/1 -> Saturation1/1, NotEqual/1  "vd_ref"
  Add8/1 -> Saturation2/1, NotEqual1/1  "vq_ref"
  vdq/1 -> Rate Transition2/1
  idq/1 -> Rate Transition3/1  "idq"
  Mux2/1 -> vdq_ref/1, Bus Creator/7  "vdq_ref"
  Demux4/2 -> Add8/1  "vq"
  Product6/1 -> [D_decoup], Add6/3  "minus_iq_L_w"
  Demux1/2 -> Add9/2  "iq"
  Product/1 -> PI_Id/1  "error"
  Demux4/1 -> Add6/1  "vd"
  Product7/1 -> Add8/3, [Q_decoup]  "id_L_w"
  Demux1/1 -> Add7/2  "id"
  Constant7/1 -> Product2/1
  Constant6/1 -> Product1/1
  PI_Id/1 -> [PId], Add6/2  "pi_id"
  Product3/1 -> PI_Iq/1  "error"
  w_pu/1 -> Rate Transition4/1

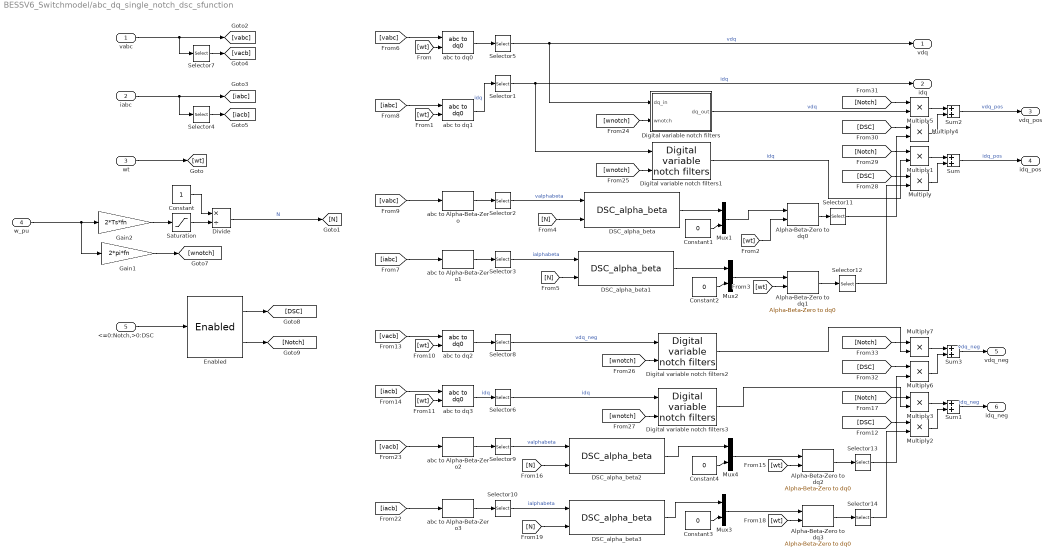
== system BESSV6_Switchmodel/abc_dq_single_notch_dsc_sfunction ==
  vabc : Inport
  iabc : Inport  Port=2
  wt : Inport  Port=3
  w_pu : Inport  Port=4
  <=0:Notch,>0:DSC : Inport  Port=5
  Alpha-Beta-Zero to dq{0..3} (4 alike) : powerlib_meascontrol/Transformations/Alpha-Beta-Zero to dq0  Alignment=90 degrees behind phase A axis
  Constant : Constant
  Constant{1..4} (4 alike) : Constant  Value=0
  DSC_alpha_beta{,1..3} (4 alike) : pwrsysBasic/DSC_alpha_beta  nmax=1/(2*Ts*fn*0.8)
      settings: SourceProductName=NTNU Power Systems
  Digital variable notch filters : Subsystem
  Digital variable notch filters1 : pwrsysTransf/abc_dq_single_notch_dsc_sfunction/Digital variable notch filters  SystemSampleTime=-1  VariantActivationTime=update diagram  Latency=0  AutoFrameSizeCalculation=off
      settings: SourceProductName=NTNU Power Systems
  Digital variable notch filters2 : pwrsysTransf/abc_dq_single_notch_dsc_sfunction/Digital variable notch filters  SystemSampleTime=-1  VariantActivationTime=update diagram  Latency=0  AutoFrameSizeCalculation=off
      settings: SourceProductName=NTNU Power Systems
  Digital variable notch filters3 : pwrsysTransf/abc_dq_single_notch_dsc_sfunction/Digital variable notch filters  SystemSampleTime=-1  VariantActivationTime=update diagram  Latency=0  AutoFrameSizeCalculation=off
      settings: SourceProductName=NTNU Power Systems
  Divide : Product  Inputs=*/
  Enabled : pwrsysBasic/Enabled
      settings: SourceProductName=NTNU Power Systems
  Gain1 : Gain  Gain=2*pi*fn
  Gain2 : Gain  Gain=2*Ts*fn
  Multiply{,1..7} (8 alike) : Product
  Mux{1..4} (4 alike) : Mux  Inputs=[2 1]
  Saturation : Saturate  UpperLimit=inf  LowerLimit=0.000001
  Selector{1..3,5..6,8..14} (12 alike) : Selector  InputPortWidth=3  IndexOptions=Index vector (dialog)  Indices=[1 2]  OutputSizes=1
  Selector4 : Selector  InputPortWidth=3  IndexOptions=Index vector (dialog)  Indices=[1 3 2]  OutputSizes=1
  Selector7 : Selector  InputPortWidth=3  IndexOptions=Index vector (dialog)  Indices=[1 3 2]  OutputSizes=1
  Sum{,1..3} (4 alike) : Sum
  abc to Alpha-Beta-Zero{,1..3} (4 alike) : powerlib_meascontrol/Transformations/abc to Alpha-Beta-Zero
  abc to dq{0..3} (4 alike) : powerlib_meascontrol/Transformations/abc to dq0  Alignment=90 degrees behind phase A axis
  vdq : Outport
  idq : Outport  Port=2
  vdq_pos : Outport  Port=3
  idq_pos : Outport  Port=4
  vdq_neg : Outport  Port=5
  idq_neg : Outport  Port=6
  wires:
  DSC_alpha_beta2/1 -> Mux4/1
  Constant4/1 -> Mux4/2
  DSC_alpha_beta3/1 -> Mux3/1
  Constant3/1 -> Mux3/2
  DSC_alpha_beta1/1 -> Mux2/1
  Constant2/1 -> Mux2/2
  Mux1/1 -> Alpha-Beta-Zero to dq0/1
  Constant1/1 -> Mux1/2
  Mux3/1 -> Alpha-Beta-Zero to dq3/1
  [wt] -> Alpha-Beta-Zero to dq3/2
  Alpha-Beta-Zero to dq3/1 -> Selector14/1
  [N] -> DSC_alpha_beta3/2
  Mux4/1 -> Alpha-Beta-Zero to dq2/1
  [wt] -> Alpha-Beta-Zero to dq2/2
  Alpha-Beta-Zero to dq2/1 -> Selector13/1
  [N] -> DSC_alpha_beta2/2
  Mux2/1 -> Alpha-Beta-Zero to dq1/1
  [wt] -> Alpha-Beta-Zero to dq1/2
  Alpha-Beta-Zero to dq1/1 -> Selector12/1
  [N] -> DSC_alpha_beta1/2
  DSC_alpha_beta/1 -> Mux1/1
  [wt] -> Alpha-Beta-Zero to dq0/2
  Alpha-Beta-Zero to dq0/1 -> Selector11/1
  abc to dq1/1 -> Selector1/1  "idq"
  Selector5/1 -> Digital variable notch filters/1(dq_in), vdq/1  "vdq"
  abc to dq0/1 -> Selector5/1
  Selector1/1 -> idq/1, Digital variable notch filters1/1  "idq"
  abc to Alpha-Beta-Zero/1 -> Selector2/1
  abc to Alpha-Beta-Zero1/1 -> Selector3/1
  Selector11/1 -> Multiply4/2
  Selector3/1 -> DSC_alpha_beta1/1  "ialphabeta"
  [vabc] -> abc to dq0/1
  [iabc] -> abc to dq1/1
  Selector2/1 -> DSC_alpha_beta/1  "valphabeta"
  Digital variable notch filters/1(dq_out) -> Multiply5/2  "vdq"
  Digital variable notch filters1/1 -> Multiply1/2  "idq"
  Selector12/1 -> Multiply/2
  Sum2/1 -> vdq_pos/1  "vdq_pos"
  Sum/1 -> idq_pos/1  "idq_pos"
  wt/1 -> [wt]
  [wt] -> abc to dq0/2
  [wt] -> abc to dq1/2
  [N] -> DSC_alpha_beta/2
  Divide/1 -> [N]  "N"
  vabc/1 -> Selector7/1, [vabc]
  Selector7/1 -> [vacb]
  iabc/1 -> Selector4/1, [iabc]
  Selector4/1 -> [iacb]
  [vabc] -> abc to Alpha-Beta-Zero/1
  [iabc] -> abc to Alpha-Beta-Zero1/1
  [wt] -> abc to dq3/2
  abc to dq2/1 -> Selector8/1
  Selector8/1 -> Digital variable notch filters2/1  "vdq_neg"
  [vacb] -> abc to dq2/1
  [wt] -> abc to dq2/2
  abc to dq3/1 -> Selector6/1  "idq"
  [iacb] -> abc to dq3/1
  Sum3/1 -> vdq_neg/1  "vdq_neg"
  Sum1/1 -> idq_neg/1  "idq_neg"
  Digital variable notch filters2/1 -> Multiply7/2
  Selector6/1 -> Digital variable notch filters3/1  "idq"
  Digital variable notch filters3/1 -> Multiply3/2
  abc to Alpha-Beta-Zero3/1 -> Selector10/1
  Selector10/1 -> DSC_alpha_beta3/1  "ialphabeta"
  abc to Alpha-Beta-Zero2/1 -> Selector9/1
  [iacb] -> abc to Alpha-Beta-Zero3/1
  [vacb] -> abc to Alpha-Beta-Zero2/1
  Selector13/1 -> Multiply6/2
  Selector9/1 -> DSC_alpha_beta2/1  "valphabeta"
  Selector14/1 -> Multiply2/2
  Gain2/1 -> Saturation/1
  Saturation/1 -> Divide/2
  Constant/1 -> Divide/1
  w_pu/1 -> Gain1/1, Gain2/1
  Gain1/1 -> [wnotch]
  [wnotch] -> Digital variable notch filters/2(wnotch)
  [wnotch] -> Digital variable notch filters1/2
  [wnotch] -> Digital variable notch filters2/2
  [wnotch] -> Digital variable notch filters3/2
  <=0:Notch,>0:DSC/1 -> Enabled/1
  Enabled/1 -> [DSC]
  Enabled/2 -> [Notch]
  [DSC] -> Multiply/1
  [Notch] -> Multiply1/1
  Multiply1/1 -> Sum/1
  Multiply/1 -> Sum/2
  [Notch] -> Multiply3/1
  [DSC] -> Multiply2/1
  Multiply3/1 -> Sum1/1
  Multiply2/1 -> Sum1/2
  [Notch] -> Multiply5/1
  Multiply4/1 -> Sum2/2
  [DSC] -> Multiply4/1
  Multiply5/1 -> Sum2/1
  [Notch] -> Multiply7/1
  Multiply6/1 -> Sum3/2
  [DSC] -> Multiply6/1
  Multiply7/1 -> Sum3/1

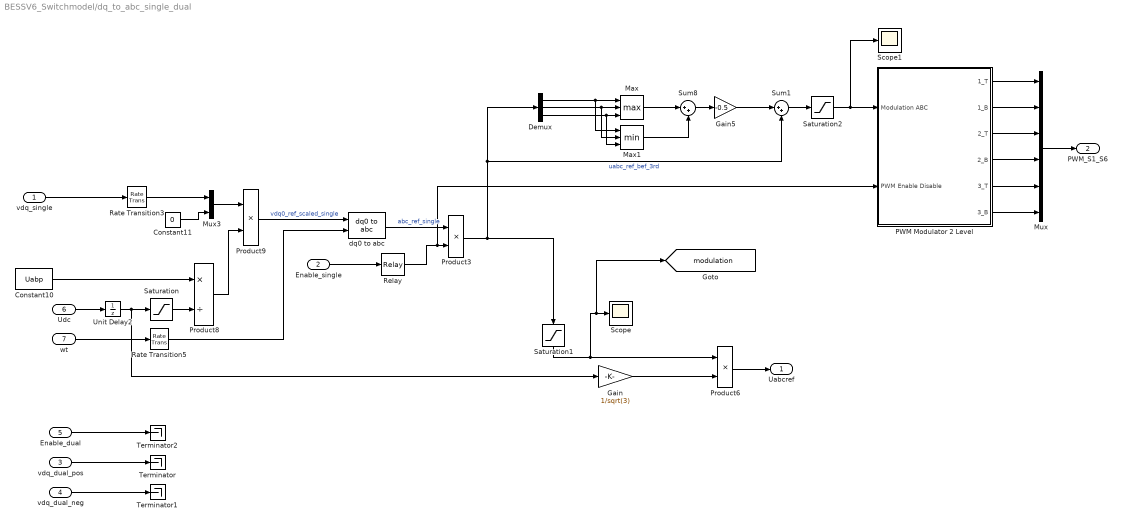
== system BESSV6_Switchmodel/dq_to_abc_single_dual ==
  vdq_single : Inport
  Enable_single : Inport  Port=2
  vdq_dual_pos : Inport  Port=3
  vdq_dual_neg : Inport  Port=4
  Enable_dual : Inport  Port=5
  Udc : Inport  Port=6
  wt : Inport  Port=7
  Constant10 : Constant  Value=Uabp  SampleTime=Ts
  Constant11 : Constant  Value=0  SampleTime=Ts
  Demux : Demux  Outputs=3
  Gain : Gain  Gain=1/sqrt(3)
  Gain5 : Gain  Gain=-0.5
  Max : MinMax  Function=max  Inputs=3
  Max1 : MinMax  Inputs=3
  Mux : Mux  Inputs=6
  Mux3 : Mux  Inputs=[2 1]
  PWM Modulator 2 Level : Subsystem
  Product3 : Product  Inputs=**
  Product6 : Product  Inputs=**
  Product8 : Product  Inputs=*/
  Product9 : Product  Inputs=**
  Rate Transition3 : RateTransition  OutPortSampleTime=Ts
  Rate Transition5 : RateTransition  OutPortSampleTime=Ts
  Relay : Relay  OnSwitchValue=0.6  OffSwitchValue=0.4
  Saturation : Saturate  UpperLimit=10*Uabp  LowerLimit=0.001*Uabp
  Saturation1 : Saturate  UpperLimit=1.0  LowerLimit=-1.0
  Saturation2 : Saturate  UpperLimit=1.0  LowerLimit=-1.0
  Scope : Scope
  Scope1 : Scope
  Sum1 : Sum  Inputs=|++
  Sum8 : Sum  Inputs=|++
  Terminator : Terminator
  Terminator1 : Terminator
  Terminator2 : Terminator
  Unit Delay2 : UnitDelay  InitialCondition=Uabp  SampleTime=Ts  HasFrameUpgradeWarning=on
  dq0 to abc : powerlib_meascontrol/Transformations/dq0 to abc  Alignment=90 degrees behind phase A axis
  Uabcref : Outport
  PWM_S1_S6 : Outport  Port=2
  tag scope: modulation=global
  wires:
  Gain/1 -> Product6/2
  Relay/1 -> PWM Modulator 2 Level/2(PWM Enable Disable), Product3/2
  Product8/1 -> Product9/2
  Saturation/1 -> Product8/2
  Product3/1 -> Saturation1/1, Sum1/2, Demux/1  "uabc_ref_bef_3rd"
  Enable_single/1 -> Relay/1
  dq0 to abc/1 -> Product3/1  "abc_ref_single"
  Constant11/1 -> Mux3/2
  Product9/1 -> dq0 to abc/1  "vdq0_ref_scaled_single"
  Unit Delay2/1 -> Saturation/1, Gain/1
  Mux3/1 -> Product9/1
  Rate Transition3/1 -> Mux3/1
  wt/1 -> Rate Transition5/1
  Constant10/1 -> Product8/1
  Udc/1 -> Unit Delay2/1
  vdq_single/1 -> Rate Transition3/1
  Product6/1 -> Uabcref/1
  Rate Transition5/1 -> dq0 to abc/2
  Saturation1/1 -> [modulation], Scope/1, Product6/1
  vdq_dual_pos/1 -> Terminator/1
  vdq_dual_neg/1 -> Terminator1/1
  Enable_dual/1 -> Terminator2/1
  Demux/1 -> Max1/1, Max/1
  Demux/2 -> Max1/2, Max/2
  Demux/3 -> Max1/3, Max/3
  Sum8/1 -> Gain5/1
  Max/1 -> Sum8/1
  Max1/1 -> Sum8/2
  Gain5/1 -> Sum1/1
  Sum1/1 -> Saturation2/1
  Saturation2/1 -> Scope1/1, PWM Modulator 2 Level/1(Modulation ABC)
  PWM Modulator 2 Level/1(1_T) -> Mux/1
  PWM Modulator 2 Level/2(1_B) -> Mux/2
  PWM Modulator 2 Level/3(2_T) -> Mux/3
  PWM Modulator 2 Level/4(2_B) -> Mux/4
  PWM Modulator 2 Level/5(3_T) -> Mux/5
  PWM Modulator 2 Level/6(3_B) -> Mux/6
  Mux/1 -> PWM_S1_S6/1

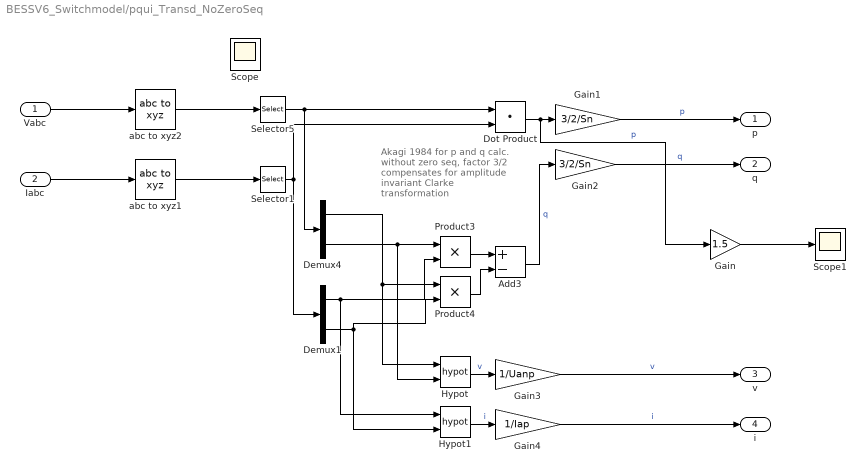
== system BESSV6_Switchmodel/pqui_Transd_NoZeroSeq ==
  note: Akagi 1984 for p and q
      | calc. without zero seq,
      | factor 3/2 compensates for
      | amplitude invariant
      | Clarke transformation
  Vabc : Inport
  Iabc : Inport  Port=2
  Add3 : Sum  Inputs=+-
  Demux1 : Demux  Outputs=2
  Demux4 : Demux  Outputs=2
  Dot Product : DotProduct  InputSameDT=on  OutDataTypeStr=Inherit: Inherit via internal rule
  Gain : Gain  Gain=1.5
  Gain1 : Gain  Gain=3/2/Sn
  Gain2 : Gain  Gain=3/2/Sn
  Gain3 : Gain  Gain=1/Uanp
  Gain4 : Gain  Gain=1/Iap
  Hypot : Math  Operator=hypot  SignedPower=on  RndMeth=Zero  SaturateOnIntegerOverflow=on
  Hypot1 : Math  Operator=hypot  SignedPower=on  RndMeth=Zero  SaturateOnIntegerOverflow=on
  Product3 : Product
  Product4 : Product
  Scope : Scope
  Scope1 : Scope
  Selector1 : Selector  InputPortWidth=3  IndexOptions=Index vector (dialog)  Indices=[1 2]  OutputSizes=1
  Selector5 : Selector  InputPortWidth=3  IndexOptions=Index vector (dialog)  Indices=[1 2]  OutputSizes=1
  abc to xyz1 : pwrsysTransf/abc to xyz  typeTransf=Amplitude-invariant
      settings: SourceProductName=NTNU Power Systems
  abc to xyz2 : pwrsysTransf/abc to xyz  typeTransf=Amplitude-invariant
      settings: SourceProductName=NTNU Power Systems
  p : Outport
  q : Outport  Port=2
  v : Outport  Port=3
  i : Outport  Port=4
  wires:
  Gain2/1 -> q/1  "q"
  Gain4/1 -> i/1  "i"
  Gain1/1 -> p/1  "p"
  Product3/1 -> Add3/1
  Iabc/1 -> abc to xyz1/1
  abc to xyz2/1 -> Selector5/1
  Vabc/1 -> abc to xyz2/1
  Demux4/2 -> Product3/1, Hypot/2
  Product4/1 -> Add3/2
  Add3/1 -> Gain2/1  "q"
  Demux1/1 -> Product3/2, Hypot1/1
  Dot Product/1 -> Gain/1, Gain1/1  "p"
  Hypot/1 -> Gain3/1  "v"
  Demux4/1 -> Hypot/1, Product4/1
  Selector5/1 -> Dot Product/1, Demux4/1
  Selector1/1 -> Dot Product/2, Demux1/1
  Hypot1/1 -> Gain4/1  "i"
  Demux1/2 -> Product4/2, Hypot1/2
  Gain3/1 -> v/1  "v"
  abc to xyz1/1 -> Selector1/1
  Gain/1 -> Scope1/1

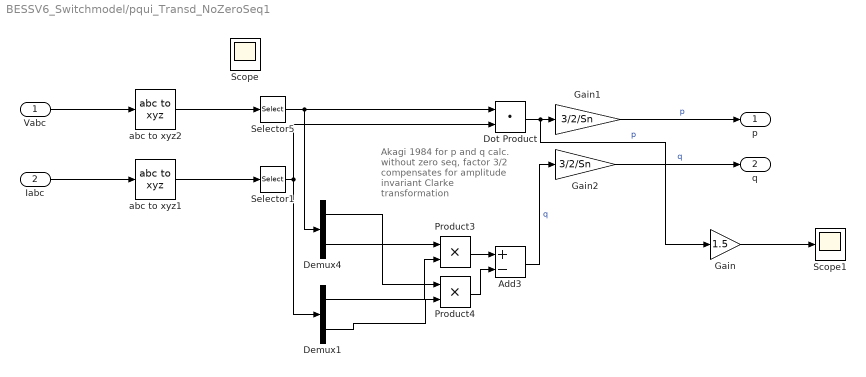
== system BESSV6_Switchmodel/pqui_Transd_NoZeroSeq1 ==
  note: Akagi 1984 for p and q
      | calc. without zero seq,
      | factor 3/2 compensates for
      | amplitude invariant
      | Clarke transformation
  Vabc : Inport
  Iabc : Inport  Port=2
  Add3 : Sum  Inputs=+-
  Demux1 : Demux  Outputs=2
  Demux4 : Demux  Outputs=2
  Dot Product : DotProduct  InputSameDT=on  OutDataTypeStr=Inherit: Inherit via internal rule
  Gain : Gain  Gain=1.5
  Gain1 : Gain  Gain=3/2/Sn
  Gain2 : Gain  Gain=3/2/Sn
  Product3 : Product
  Product4 : Product
  Scope : Scope
  Scope1 : Scope
  Selector1 : Selector  InputPortWidth=3  IndexOptions=Index vector (dialog)  Indices=[1 2]  OutputSizes=1
  Selector5 : Selector  InputPortWidth=3  IndexOptions=Index vector (dialog)  Indices=[1 2]  OutputSizes=1
  abc to xyz1 : pwrsysTransf/abc to xyz  typeTransf=Amplitude-invariant
      settings: SourceProductName=NTNU Power Systems
  abc to xyz2 : pwrsysTransf/abc to xyz  typeTransf=Amplitude-invariant
      settings: SourceProductName=NTNU Power Systems
  p : Outport
  q : Outport  Port=2
  wires:
  Gain2/1 -> q/1  "q"
  Gain1/1 -> p/1  "p"
  Product3/1 -> Add3/1
  Iabc/1 -> abc to xyz1/1
  abc to xyz2/1 -> Selector5/1
  Vabc/1 -> abc to xyz2/1
  Demux4/2 -> Product3/1
  Product4/1 -> Add3/2
  Add3/1 -> Gain2/1  "q"
  Demux1/1 -> Product3/2
  Dot Product/1 -> Gain/1, Gain1/1  "p"
  Demux4/1 -> Product4/1
  Selector5/1 -> Dot Product/1, Demux4/1
  Selector1/1 -> Dot Product/2, Demux1/1
  Demux1/2 -> Product4/2
  abc to xyz1/1 -> Selector1/1
  Gain/1 -> Scope1/1

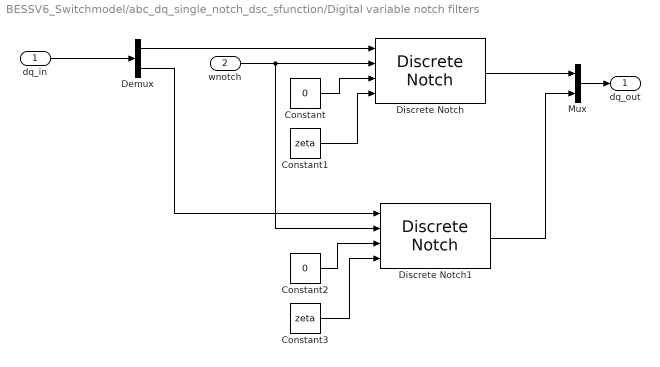
== system BESSV6_Switchmodel/abc_dq_single_notch_dsc_sfunction/Digital variable notch filters ==
  dq_in : Inport
  wnotch : Inport  Port=2
  Constant : Constant  Value=0
  Constant1 : Constant  Value=zeta
  Constant2 : Constant  Value=0
  Constant3 : Constant  Value=zeta
  Demux : Demux  Outputs=2
  Discrete Notch : pwrsysBasic/Discrete Notch  Ts=Ts
      settings: SourceProductName=NTNU Power Systems
  Discrete Notch1 : pwrsysBasic/Discrete Notch  Ts=Ts
      settings: SourceProductName=NTNU Power Systems
  Mux : Mux  Inputs=2
  dq_out : Outport
  wires:
  Demux/2 -> Discrete Notch1/1
  dq_in/1 -> Demux/1
  Constant2/1 -> Discrete Notch1/3
  wnotch/1 -> Discrete Notch/2, Discrete Notch1/2
  Constant3/1 -> Discrete Notch1/4
  Mux/1 -> dq_out/1
  Discrete Notch1/1 -> Mux/2
  Demux/1 -> Discrete Notch/1
  Constant/1 -> Discrete Notch/3
  Constant1/1 -> Discrete Notch/4
  Discrete Notch/1 -> Mux/1

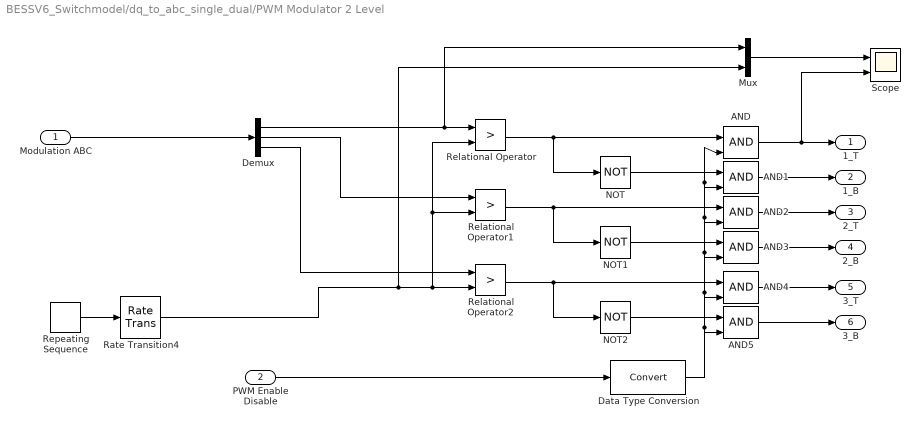
== system BESSV6_Switchmodel/dq_to_abc_single_dual/PWM Modulator 2 Level ==
  Modulation ABC : Inport
  PWM Enable Disable : Inport  Port=2
  AND{,1..5} (6 alike) : Logic  IconShape=distinctive  AllPortsSameDT=off  OutDataTypeStr=boolean
  Data Type Conversion : DataTypeConversion
  Demux : Demux  Outputs=3
  Mux : Mux  Inputs=2
  NOT : Logic  Operator=NOT  IconShape=distinctive  AllPortsSameDT=off  OutDataTypeStr=boolean
  NOT1 : Logic  Operator=NOT  IconShape=distinctive  AllPortsSameDT=off  OutDataTypeStr=boolean
  NOT2 : Logic  Operator=NOT  IconShape=distinctive  AllPortsSameDT=off  OutDataTypeStr=boolean
  Rate Transition4 : RateTransition  OutPortSampleTime=ess.Ts_control
  Relational Operator : RelationalOperator  Operator=>  OutDataTypeStr=boolean  RndMeth=Simplest
  Relational Operator1 : RelationalOperator  Operator=>  OutDataTypeStr=boolean  RndMeth=Simplest
  Relational Operator2 : RelationalOperator  Operator=>  OutDataTypeStr=boolean  RndMeth=Simplest
  Repeating Sequence : simulink/Sources/Repeating Sequence  rep_seq_t=[0 1 2 3 4]*(ess.Tsw/4)  rep_seq_y=[0 1 0 -1 0]
  Scope : Scope  NumInputPorts=2
  1_T : Outport
  1_B : Outport  Port=2
  2_T : Outport  Port=3
  2_B : Outport  Port=4
  3_T : Outport  Port=5
  3_B : Outport  Port=6
  wires:
  Data Type Conversion/1 -> AND5/2, AND4/2, AND3/2, AND2/2, AND1/2, AND/2
  Relational Operator2/1 -> AND4/1, NOT2/1
  AND2/1 -> 2_T/1
  PWM Enable Disable/1 -> Data Type Conversion/1
  Relational Operator/1 -> AND/1, NOT/1
  NOT/1 -> AND1/1
  Relational Operator1/1 -> AND2/1, NOT1/1
  NOT1/1 -> AND3/1
  NOT2/1 -> AND5/1
  AND4/1 -> 3_T/1
  AND3/1 -> 2_B/1
  AND5/1 -> 3_B/1
  AND1/1 -> 1_B/1
  AND/1 -> Scope/2, 1_T/1
  Demux/1 -> Mux/1, Relational Operator/1
  Demux/2 -> Relational Operator1/1
  Demux/3 -> Relational Operator2/1
  Modulation ABC/1 -> Demux/1
  Mux/1 -> Scope/1
  Repeating Sequence/1 -> Rate Transition4/1
  Rate Transition4/1 -> Mux/2, Relational Operator/2, Relational Operator1/2, Relational Operator2/2
